simulink model "OPC_GreenCrane"  (R2024b)
settings: Solver=FixedStepDiscrete  StartTime=0.0  StopTime=inf  FixedStep=0.01  MaxStep=0.001  RelTol=1e-3
libraries: opcualib x1, sldrtlib x1
settings Model: Creator=Green Crane Testbed  LastModifiedBy=Green Crane Testbed

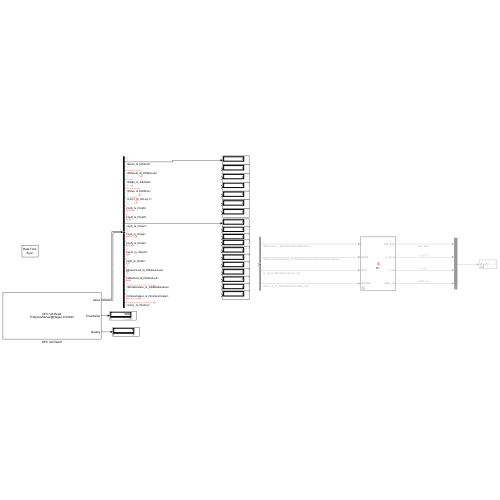
[thumbnail: Simulink's stored preview of the top-level diagram]
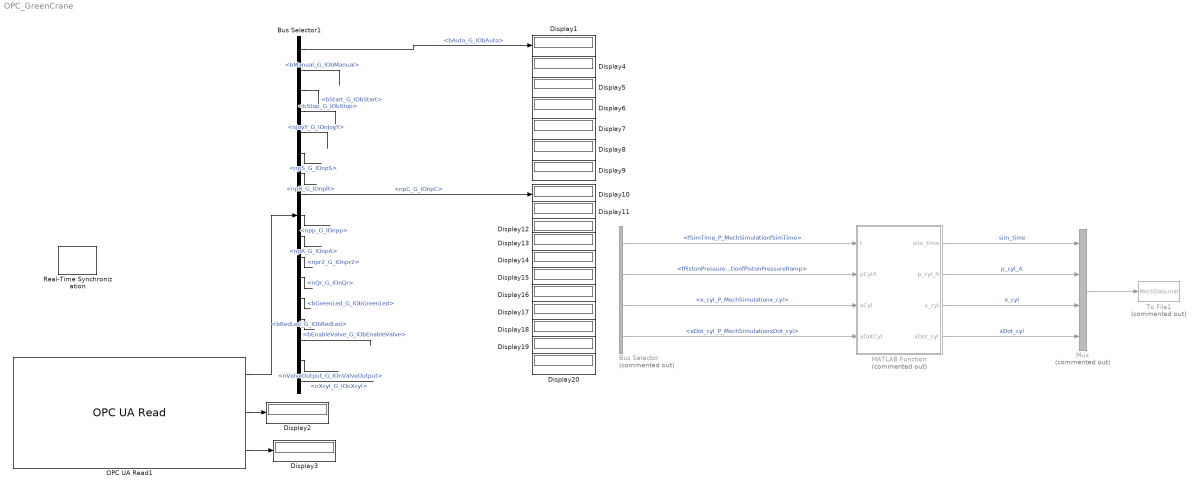
== system OPC_GreenCrane ==
  Bus Selector : BusSelector  Commented=on  OutputSignals=fSimTime_P_MechSimulationfSimTime,fPistonPressureRamp_P_MechSimulationfPistonPressureRamp,x_cyl_P_MechSimulationx_cyl,xDot_cyl_P_MechSimulationxDot_cyl
  Bus Selector1 : BusSelector  OutputSignals=bAuto_G_IObAuto,bManual_G_IObManual,bStart_G_IObStart,bStop_G_IObStop,nJoyY_G_IOnJoyY,npS_G_IOnpS,npR_G_IOnpR,npC_G_IOnpC,npp_G_IOnpp,npA_G_IOnpA,npr2_G_IOnpr2,nQr_G_IOnQr,bGreenLed_G_IObGreenLed,bRedLed_G_IObRedLed,bEnableValve_G_IObEnableValve,nValveOutput_G_IOnValveOutput,nXcyl_G_IOnXcyl
  Display{1..20} (20 alike) : Display
  MATLAB Function : MATLAB Function  Commented=on  TreatAsAtomicUnit=on
  Mux : Mux  Commented=on
  OPC UA Read1 : opcualib/OPC UA Read  SelectedServer=TcOpcUaServer@Hagen-CX2043  ServerList=TcOpcUaServer@Hagen-CX2043  NodeList={ '1', 'bAuto', '4', 'G_IO.bAuto', '0'; '2', 'bManual', '4', 'G_IO.bManual', '0'; '3', 'bStart', '4', 'G_IO.bStart', '0'; '4', 'bStop', '4', 'G_IO.bStop', '0'; '5', 'nJoyY', '4', 'G_IO.nJoyY', '0'; '6', 'npS', '4', 'G_IO.npS', '0'; '7', 'npR', '4', 'G_IO.npR', '0'; '8', 'npC', '4', 'G_IO.npC', '0'; '9', 'npp', '4', 'G_IO.npp', '0'; '10', 'npA', '4', 'G_IO.npA', '0'; '11', 'npr2', '4', 'G_IO.npr2', '0'; '12', 'nQr', '4', 'G_IO.nQr', '0'; '13', 'bGreenLed', '4', 'G_IO.bGreenLed', '0'; '14', 'bRedLed', '4', 'G_IO.bRedLed', '0'; '15', 'bEnableValve', '4', 'G_IO.bEnableValve', '0'; '16', 'nValveOutput', '4', 'G_IO.nValveOutput', '0'; '17', 'nXcyl', '4', 'G_IO.nXcyl', '0' }  ShowQualityPort=on  ShowTimestampPort=on  ShowTimestampPortAs=Seconds since start  SampleTime=-1
  Real-Time Synchronization : sldrtlib/Real-Time Synchronization  SampleTime=-1  MaxMissedTicks=1000000000000  ShowMissedTicks=off  YieldWhenWaiting=off
  To File1 : ToFile  Commented=on  Filename=MechData.mat  SaveFormat=Timeseries
  wires:
  Bus Selector/1 -> MATLAB Function/1(t)  "<fSimTime_P_MechSimulationfSimTime>"
  Bus Selector/2 -> MATLAB Function/2(pCylA)  "<fPistonPressureRamp_P_MechSimulationfPistonPressureRamp>"
  Bus Selector/3 -> MATLAB Function/3(xCyl)  "<x_cyl_P_MechSimulationx_cyl>"
  Bus Selector/4 -> MATLAB Function/4(xDotCyl)  "<xDot_cyl_P_MechSimulationxDot_cyl>"
  MATLAB Function/1(sim_time) -> Mux/1  "sim_time"
  MATLAB Function/2(p_cyl_A) -> Mux/2  "p_cyl_A"
  MATLAB Function/3(x_cyl) -> Mux/3  "x_cyl"
  MATLAB Function/4(xDot_cyl) -> Mux/4  "xDot_cyl"
  Mux/1 -> To File1/1
  OPC UA Read1/1 -> Bus Selector1/1
  OPC UA Read1/3 -> Display3/1
  OPC UA Read1/2 -> Display2/1
  Bus Selector1/1 -> Display1/1  "<bAuto_G_IObAuto>"
  Bus Selector1/15 -> ?  "<bEnableValve_G_IObEnableValve>"
  Bus Selector1/16 -> ?  "<nValveOutput_G_IOnValveOutput>"
  Bus Selector1/14 -> ?  "<bRedLed_G_IObRedLed>"
  Bus Selector1/13 -> ?  "<bGreenLed_G_IObGreenLed>"
  Bus Selector1/12 -> ?  "<nQr_G_IOnQr>"
  Bus Selector1/11 -> ?  "<npr2_G_IOnpr2>"
  Bus Selector1/10 -> ?  "<npA_G_IOnpA>"
  Bus Selector1/9 -> ?  "<npp_G_IOnpp>"
  Bus Selector1/8 -> Display10/1  "<npC_G_IOnpC>"
  Bus Selector1/7 -> ?  "<npR_G_IOnpR>"
  Bus Selector1/6 -> ?  "<npS_G_IOnpS>"
  Bus Selector1/5 -> ?  "<nJoyY_G_IOnJoyY>"
  Bus Selector1/4 -> ?  "<bStop_G_IObStop>"
  Bus Selector1/3 -> ?  "<bStart_G_IObStart>"
  Bus Selector1/2 -> ?  "<bManual_G_IObManual>"
  Bus Selector1/17 -> ?  "<nXcyl_G_IOnXcyl>"

== matlab function OPC_GreenCrane/MATLAB Function ==
  data: t input; sim_time output; p_cyl_A output; x_cyl output; xDot_cyl output; pCylA input; xCyl input; xDotCyl input
function [sim_time, p_cyl_A, x_cyl, xDot_cyl]   = fcn(t, pCylA, xCyl, xDotCyl)
if t >= 0.0 && t < 10.0
     sim_time = t;
     p_cyl_A = pCylA;
     x_cyl = xCyl;
     xDot_cyl = xDotCyl;
elseif t >= 10.0
     sim_time = 10.0;
     p_cyl_A = pCylA;
     x_cyl = xCyl;
     xDot_cyl = xDotCyl;
else
     sim_time = 0.0;
     p_cyl_A = 0.0;
     x_cyl = 0.0;
     xDot_cyl = 0.0;
end
